simulink model "Subsystem"  (R2020b)
settings: Solver=VariableStepAuto  StartTime=0.0  StopTime=10.0  RelTol=1e-3
settings Model: Creator=Sudhanshu  LastModifiedBy=Sudhanshu
settings DataIOCC: SaveOutput=off  SaveTime=off

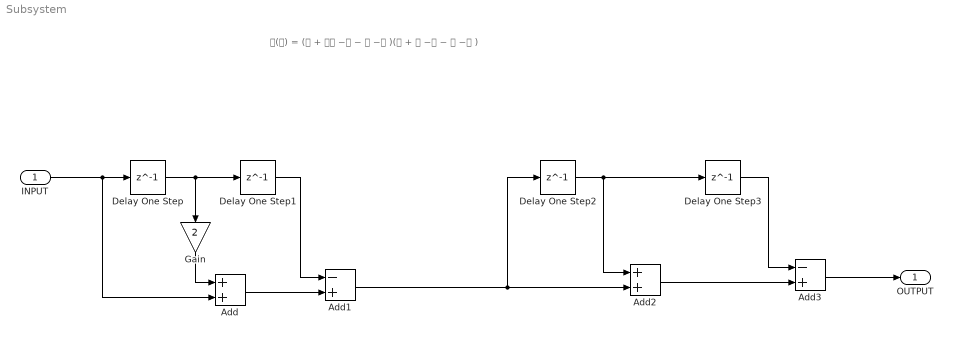
== system Subsystem ==
  note: 𝐇(𝐳) = (𝟏 + 𝟐𝐳 −𝟏 − 𝐳 −𝟐 )(𝟏 + 𝐳 −𝟏 − 𝐳 −𝟐 )
  INPUT : Inport  OutDataTypeStr=double  PortDimensions=1  SampleTime=[0,1]
  Add : Sum
  Add1 : Sum  Inputs=-+
  Add2 : Sum
  Add3 : Sum  Inputs=-+
  Delay One Step{,1..3} (4 alike) : Delay  DelayLength=1
  Gain : Gain  Gain=2
  OUTPUT : Outport  OutDataTypeStr=double  PortDimensions=1  SampleTime=[0,1]
  wires:
  Add2/1 -> Add3/2
  Gain/1 -> Add/1
  Delay One Step/1 -> Delay One Step1/1, Gain/1
  INPUT/1 -> Delay One Step/1, Add/2
  Add/1 -> Add1/2
  Delay One Step2/1 -> Add2/1, Delay One Step3/1
  Delay One Step1/1 -> Add1/1
  Delay One Step3/1 -> Add3/1
  Add1/1 -> Add2/2, Delay One Step2/1
  Add3/1 -> OUTPUT/1
